simulink model "mdl_K"  (Simulink 4.00)
settings: Solver=ode45  StartTime=0.0  StopTime=15  RelTol=1e-3
values from neighbouring files (symbols this model uses):
  A = [ -0.5  0  0;  0  -2  10;  0  1  -2 ]    [st_KS_minMax.m]
  B = [ 1  0;  -2  2;  0  1 ]    [st_KS_minMax.m]
  C = [ 1  0  0;  0  0  1 ]    [st_KS_minMax.m]
  K = [RGenes(1:2); RGenes(3:4)]    [st_KS_minMax.m]
undefined symbols (not defined in the file or in its folder): sfunyst
settings Model: LastModifiedBy=LPEE_Plamen  BlockReductionOpt=off

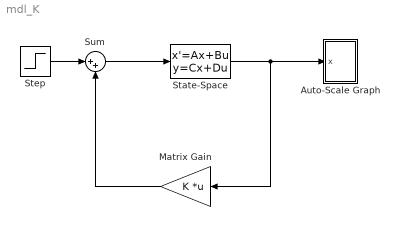
== system mdl_K ==
  Auto-Scale Graph : Subsystem  mask(Storage scope.){@1=5, @2=0, @3=10, @4=2000, @5='r-/b-/c-/k-/m*/ro/b+'}
      mask prompts: @1 "Initial Time Range:"; @2 "Initial y-min:"; @3 "Initial y-max:"; @4 "Storage pts.:"; @5 "Line type (rgbw-.:xo):"
      mask help:
      | Storage scope using MATLAB graph window.
      | Enter plotting ranges and line type.
      mask init:
      | npts = @4; color = @5; ax = [0, @1, @2, @3]; dt=-1;
      settings: RTWFcnNameOpts=Auto  RTWFileNameOpts=Auto
      mask Help: This block uses a MATLAB figure window to plot the input signal.  The graph limits are automatically scaled to the min and max values of the signal stored in the scope's signal buffer.  Line type must be in quotes.  See the M-file sfunyst.m.
      mask Display: plot(0,0,100,100,[83,76,63,52,42,38,28,16,11,84,11,11,11,90,90,11],[75,58,47,54,72,80,84,74,65,65,65,90,40,40,90,90])
  Matrix Gain : Gain  Orientation=left  Gain=K  Multiplication=Matrix(K*u)  SaturateOnIntegerOverflow=on
  State-Space : StateSpace  A=A  B=B  C=C  D=[ 0 0; 0 0 ]  X0=0  Realization=auto  AbsoluteTolerance=auto
  Step : Step  Time=0  Before=0  After=1  SampleTime=0
  Sum : Sum  Inputs=|++  SaturateOnIntegerOverflow=on
  wires:
  Step/1 -> Sum/1
  Sum/1 -> State-Space/1
  State-Space/1 -> Auto-Scale Graph/1(x), Matrix Gain/1
  Matrix Gain/1 -> Sum/2

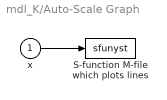
== system mdl_K/Auto-Scale Graph ==
  x : Inport  Port=1
  "S-function M-file which plots lines " : S-Function  LoadFcn=sfunyst([],[],[],'LoadBlock')  FunctionName=sfunyst  Parameters=ax, color, npts, dt  PortCounts=[]  SFunctionModules=''
      settings: CopyFcn=sfunyst([],[],[],'CopyBlock')  DeleteFcn=sfunyst([],[],[],'DeleteBlock')
  wires:
  x/1 -> "S-function M-file which plots lines "/1
